simulink model "Rocket_model_Stateflow_testing"  (R2022b)
settings: Solver=VariableStepAuto  StartTime=0.0  StopTime=500  RelTol=1e-3
values from neighbouring files (symbols this model uses):
  GSE_Pipe_Cross_sectional_Area = 7.48    [Rocket_gas_model_setting.m]
  GSE_Pipe_Hydr_Diameter = 2.1    [Rocket_gas_model_setting.m]
  Hose_length = 2    [Rocket_gas_model_setting.m]
  N2_Gas_Tank_Diameter = 0.229    [Rocket_gas_model_setting.m]
  N2_Gas_Tank_Height = 0.5    [Rocket_gas_model_setting.m]
  N2_Rocket_Tank_Diameter = 0.146    [Rocket_gas_model_setting.m]
  N2_Rocket_Tank_Height = 1.515    [Rocket_gas_model_setting.m]
  Outside_temperature = 20    [Rocket_gas_model_setting.m]
  Rocket_Pipe_Cross_sectional_Area = 2    [Rocket_gas_model_setting.m]
  Rocket_Pipe_Hydr_Diameter = 4    [Rocket_gas_model_setting.m]
  s = struct    [State_Flow_varB_setting.m]
libraries: fl_lib x48, nesl_utility x10, slrealtimeiplib x5
settings Model: Creator=START  LastModifiedBy=START

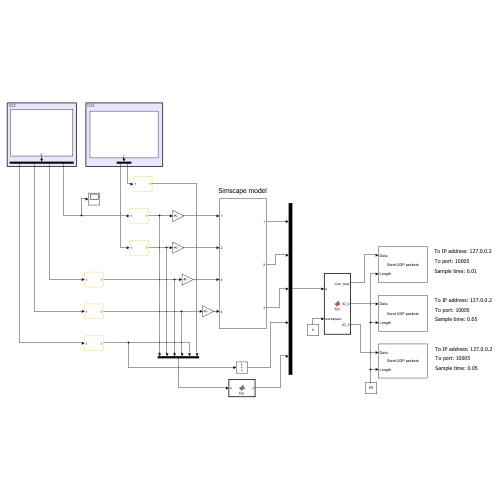
[thumbnail: Simulink's stored preview of the top-level diagram]
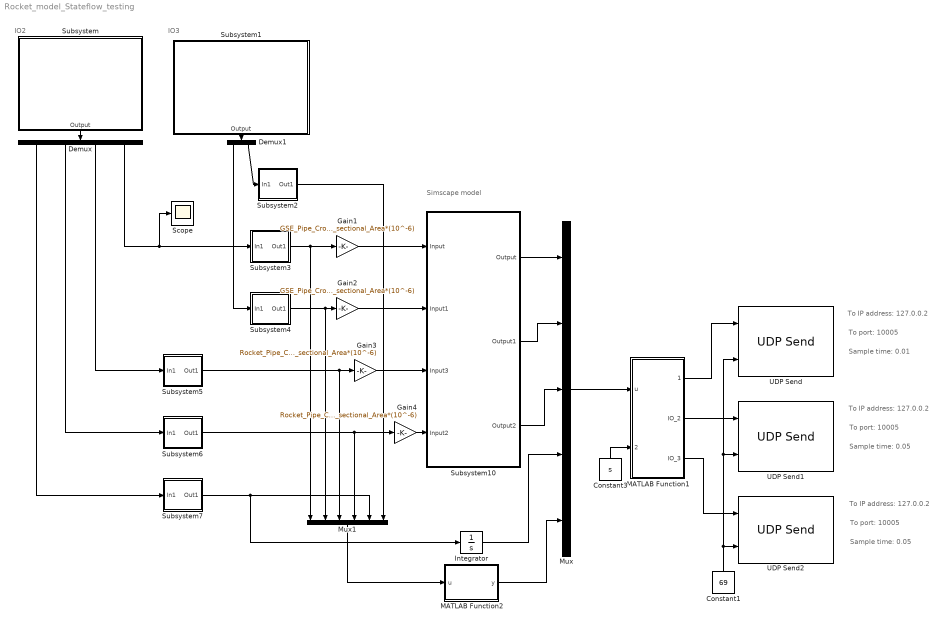
== system Rocket_model_Stateflow_testing ==
  note: Simscape model
  note: To port: 10005
  note: To IP address: 127.0.0.2
  note: IO2
  note: IO3
  note: Sample time: 0.01
  note: Sample time: 0.05
  note: To IP address: 127.0.0.2
  note: To port: 10005
  note: Sample time: 0.05
  note: To IP address: 127.0.0.2
  note: To port: 10005
  Constant1 : Constant  Value=69
  Constant3 : Constant  Value=s  OutDataTypeStr=Bus: s_bus
  Demux : Demux
  Demux1 : Demux  Outputs=2
  Gain1 : Gain  Gain=GSE_Pipe_Cross_sectional_Area*(10^-6)
  Gain2 : Gain  Gain=GSE_Pipe_Cross_sectional_Area*(10^-6)
  Gain3 : Gain  Gain=Rocket_Pipe_Cross_sectional_Area*(10^-6)
  Gain4 : Gain  Gain=Rocket_Pipe_Cross_sectional_Area*(10^-6)
  Integrator : Integrator
  MATLAB Function1 : MATLAB Function  TreatAsAtomicUnit=on
  MATLAB Function2 : MATLAB Function  TreatAsAtomicUnit=on
  Mux : Mux  Inputs=5
  Mux1 : Mux  Inputs=6
  Scope : Scope
  Subsystem : Subsystem
  Subsystem1 : Subsystem
  Subsystem10 : Subsystem
  Subsystem2 : Subsystem
  Subsystem3 : Subsystem
  Subsystem4 : Subsystem
  Subsystem5 : Subsystem
  Subsystem6 : Subsystem
  Subsystem7 : Subsystem
  UDP Send : slrealtimeiplib/UDP Send  useHostTargetConn=off  toAddress=UDP_GSE_receive_local_IP  toPort=UDP_GSE_receive_local_PORT  sampleTime=UDP_GSE_Curr_loop_receive_sample_time  enableMessage=off
  UDP Send1 : slrealtimeiplib/UDP Send  useHostTargetConn=off  toAddress=UDP_GSE_receive_local_IP  toPort=UDP_GSE_receive_local_PORT  sampleTime=UDP_GSE_IO_receive_sample_time  enableMessage=off
  UDP Send2 : slrealtimeiplib/UDP Send  useHostTargetConn=off  toAddress=UDP_GSE_receive_local_IP  toPort=UDP_GSE_receive_local_PORT  sampleTime=UDP_GSE_IO_receive_sample_time  enableMessage=off
  wires:
  Subsystem10/1(Output) -> Mux/1
  Subsystem10/2(Output1) -> Mux/2
  Mux/1 -> MATLAB Function1/1(u)
  Constant1/1 -> UDP Send1/2, UDP Send/2, UDP Send2/2
  Subsystem10/3(Output2) -> Mux/3
  Demux/3 -> Subsystem5/1(In1)
  Subsystem3/1(Out1) -> Gain1/1, Mux1/1
  Subsystem4/1(Out1) -> Gain2/1, Mux1/2
  Subsystem5/1(Out1) -> Gain3/1, Mux1/3
  Demux/2 -> Subsystem6/1(In1)
  Constant3/1 -> MATLAB Function1/2(workspace)
  Subsystem6/1(Out1) -> Gain4/1, Mux1/4
  MATLAB Function2/1(y) -> Mux/5
  Mux1/1 -> MATLAB Function2/1(u)
  MATLAB Function1/1(Curr_loop) -> UDP Send/1
  MATLAB Function1/2(IO_2) -> UDP Send1/1
  MATLAB Function1/3(IO_3) -> UDP Send2/1
  Subsystem7/1(Out1) -> Mux1/5, Integrator/1
  Integrator/1 -> Mux/4
  Subsystem/1(Output) -> Demux/1
  Demux/1 -> Subsystem7/1(In1)
  Demux/4 -> Scope/1, Subsystem3/1(In1)
  Subsystem1/1(Output) -> Demux1/1
  Demux1/1 -> Subsystem4/1(In1)
  Demux1/2 -> Subsystem2/1(In1)
  Subsystem2/1(Out1) -> Mux1/6
  Gain1/1 -> Subsystem10/1(Input)
  Gain2/1 -> Subsystem10/2(Input1)
  Gain3/1 -> Subsystem10/3(Input3)
  Gain4/1 -> Subsystem10/4(Input2)

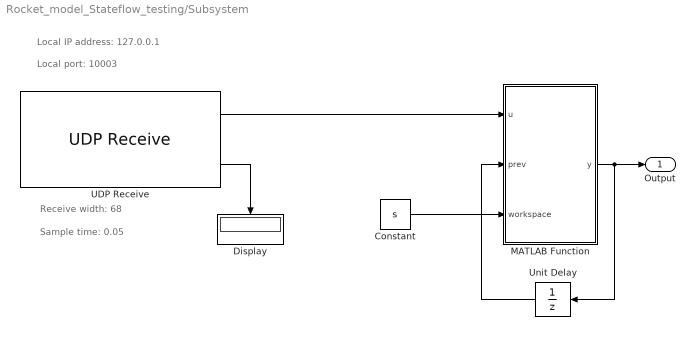
== system Rocket_model_Stateflow_testing/Subsystem ==
  note: Local IP address: 127.0.0.1
  note: Local port: 10003
  note: Receive width: 68
  note: Sample time: 0.05
  Constant : Constant  Value=s  OutDataTypeStr=Bus: s_bus
  Display : Display
  MATLAB Function : MATLAB Function  TreatAsAtomicUnit=on
  UDP Receive : slrealtimeiplib/UDP Receive  useHostTargetConn=off  ipAddress=UDP_GSE_send_to_IP  localPort=IO_card_2_port  rcvWidth=UDP_GSE_send_packet_length  rcvFmAny=on  fmAddress='10.10.10.10'  sampleTime=UDP_GSE_IO_receive_sample_time  enableMessage=off  maxPackets=1
  Unit Delay : UnitDelay  SampleTime=-1  HasFrameUpgradeWarning=on
  Output : Outport
  wires:
  UDP Receive/1 -> MATLAB Function/1(u)
  MATLAB Function/1(y) -> Output/1, Unit Delay/1
  Constant/1 -> MATLAB Function/3(workspace)
  UDP Receive/2 -> Display/1
  Unit Delay/1 -> MATLAB Function/2(prev)

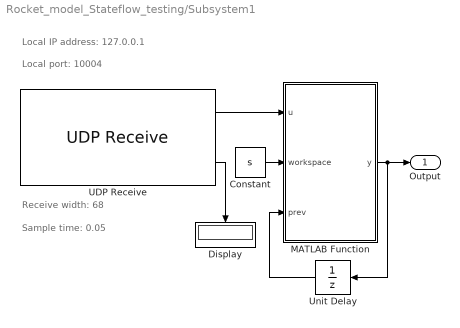
== system Rocket_model_Stateflow_testing/Subsystem1 ==
  note: Local IP address: 127.0.0.1
  note: Local port: 10004
  note: Receive width: 68
  note: Sample time: 0.05
  Constant : Constant  Value=s  OutDataTypeStr=Bus: s_bus
  Display : Display
  MATLAB Function : MATLAB Function  TreatAsAtomicUnit=on
  UDP Receive : slrealtimeiplib/UDP Receive  useHostTargetConn=off  ipAddress=UDP_GSE_send_to_IP  localPort=IO_card_3_port  rcvWidth=UDP_GSE_send_packet_length  rcvFmAny=on  fmAddress='10.10.10.10'  sampleTime=UDP_GSE_IO_receive_sample_time  enableMessage=off  maxPackets=1
  Unit Delay : UnitDelay  InitialCondition=[0,0]  SampleTime=-1  HasFrameUpgradeWarning=on
  Output : Outport
  wires:
  UDP Receive/1 -> MATLAB Function/1(u)
  MATLAB Function/1(y) -> Output/1, Unit Delay/1
  Constant/1 -> MATLAB Function/2(workspace)
  UDP Receive/2 -> Display/1
  Unit Delay/1 -> MATLAB Function/3(prev)

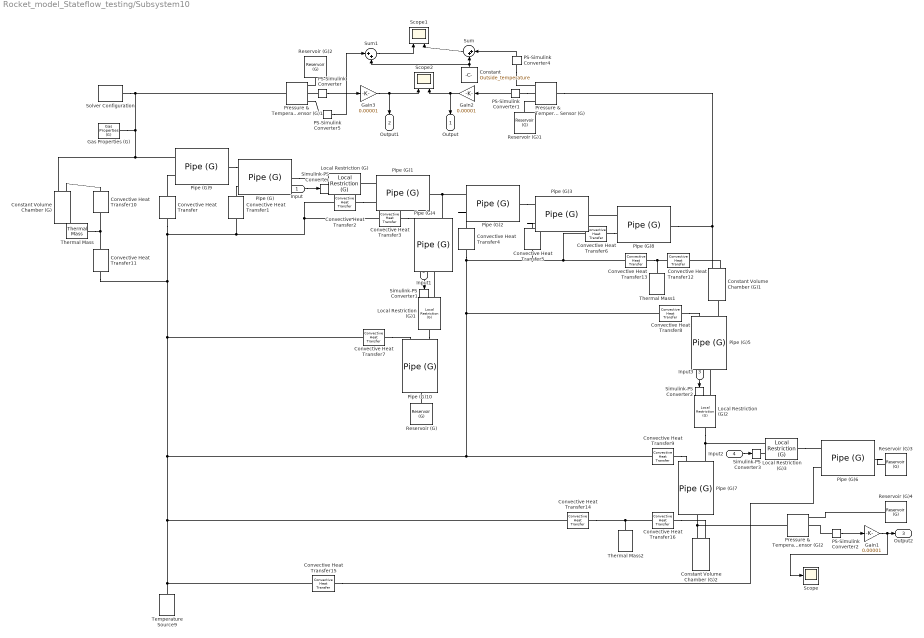
== system Rocket_model_Stateflow_testing/Subsystem10 ==
  Input : Inport
  Input1 : Inport  Port=2
  Input3 : Inport  Port=3
  Input2 : Inport  Port=4
  Constant : Constant  Value=Outside_temperature
  Constant Volume Chamber (G) : fl_lib/Gas/Elements/Constant Volume Chamber (G)  volume=N2_Gas_Tank_Volume m^3  num_ports=foundation.enum.num_ports.one  area_A=0.001 m^2  area_B=0.01 m^2  area_C=0.01 m^2  area_D=0.01 m^2  p_I_specify=on  p_I_priority=High  p_I=N2_Gas_Tank_Pressure bar  p_I_nominal_specify=off  p_I_nominal_unit=MPa  p_I_nominal_value=1  T_I_specify=on  T_I_priority=Low  T_I=Outside_temperature degC  T_I_nominal_specify=off  T_I_nominal_unit=K  T_I_nominal_value=293  rho_chamber_specify=off  rho_chamber_priority=None  rho_chamber=1.2 kg/m^3  rho_chamber_nominal_specify=off  rho_chamber_nominal_unit=kg/m^3  rho_chamber_nominal_value=1
      settings: InternalSimscapePortConfiguration="{\"Bottom\":[],\"Left\":[{\"id\":\"A\",\"label\":\"A\",\"type\":\"foundation.gas.gas\"},{\"id\":\"H\",\"label\":\"H\",\"type\":\"foundation.thermal.thermal\"}],\"Right\":[],\"Top\":[]}"
  Constant Volume Chamber (G)1 : fl_lib/Gas/Elements/Constant Volume Chamber (G)  volume=N2_Rocket_Tank_Volume m^3  num_ports=foundation.enum.num_ports.two  area_A=0.001 m^2  area_B=0.001 m^2  area_C=0.01 m^2  area_D=0.01 m^2  p_I_specify=on  p_I_priority=High  p_I=1 bar  p_I_nominal_specify=off  p_I_nominal_unit=MPa  p_I_nominal_value=1  T_I_specify=on  T_I_priority=Low  T_I=Outside_temperature degC  T_I_nominal_specify=off  T_I_nominal_unit=K  T_I_nominal_value=320  rho_chamber_specify=off  rho_chamber_priority=None  rho_chamber=1.2 kg/m^3  rho_chamber_nominal_specify=off  rho_chamber_nominal_unit=kg/m^3  rho_chamber_nominal_value=1
      settings: InternalSimscapePortConfiguration="{\"Bottom\":[],\"Left\":[{\"id\":\"A\",\"label\":\"A\",\"type\":\"foundation.gas.gas\"},{\"id\":\"H\",\"label\":\"H\",\"type\":\"foundation.thermal.thermal\"}],\"Right\":[{\"id\":\"B\",\"label\":\"B\",\"type\":\"foundation.gas.gas\"}],\"Top\":[]}"
  Constant Volume Chamber (G)2 : fl_lib/Gas/Elements/Constant Volume Chamber (G)  volume=N2O_Rocket_Tank_Volume m^3  num_ports=foundation.enum.num_ports.one  area_A=0.001 m^2  area_B=0.001 m^2  area_C=0.01 m^2  area_D=0.01 m^2  p_I_specify=on  p_I_priority=High  p_I=1 bar  p_I_nominal_specify=off  p_I_nominal_unit=MPa  p_I_nominal_value=1  T_I_specify=on  T_I_priority=Low  T_I=Outside_temperature degC  T_I_nominal_specify=off  T_I_nominal_unit=K  T_I_nominal_value=320  rho_chamber_specify=off  rho_chamber_priority=None  rho_chamber=1.2 kg/m^3  rho_chamber_nominal_specify=off  rho_chamber_nominal_unit=kg/m^3  rho_chamber_nominal_value=1
      settings: InternalSimscapePortConfiguration="{\"Bottom\":[],\"Left\":[{\"id\":\"A\",\"label\":\"A\",\"type\":\"foundation.gas.gas\"},{\"id\":\"H\",\"label\":\"H\",\"type\":\"foundation.thermal.thermal\"}],\"Right\":[],\"Top\":[]}"
  Convective Heat Transfer : fl_lib/Thermal/Thermal Elements/Convective Heat Transfer  thermal_type=foundation.enum.constant_variable.constant  area=GSE_Pipe_Hydr_Diameter*(Hose_length*1000) mm^2  heat_tr_coeff=15 W/(K*m^2)  min_heat_tr_coeff=1e-3 W/(K*m^2)  T_specify=off  T_priority=None  T=0 K  T_nominal_specify=off  T_nominal_unit=K  T_nominal_value=1  Q_specify=off  Q_priority=None  Q=0 W  Q_nominal_specify=off  Q_nominal_unit=W  Q_nominal_value=1
  Convective Heat Transfer1 : fl_lib/Thermal/Thermal Elements/Convective Heat Transfer  thermal_type=foundation.enum.constant_variable.constant  area=GSE_Pipe_Hydr_Diameter*(0.3*1000) mm^2  heat_tr_coeff=15 W/(K*m^2)  min_heat_tr_coeff=1e-3 W/(K*m^2)  T_specify=off  T_priority=None  T=0 K  T_nominal_specify=off  T_nominal_unit=K  T_nominal_value=1  Q_specify=off  Q_priority=None  Q=0 W  Q_nominal_specify=off  Q_nominal_unit=W  Q_nominal_value=1
  Convective Heat Transfer10 : fl_lib/Thermal/Thermal Elements/Convective Heat Transfer  thermal_type=foundation.enum.constant_variable.constant  area="N2_Gas_Tank_Diameter*N2_Gas_Tank_Height  m^2"  heat_tr_coeff=15 W/(K*m^2)  min_heat_tr_coeff=1e-3 W/(K*m^2)  T_specify=off  T_priority=None  T=0 K  T_nominal_specify=off  T_nominal_unit=K  T_nominal_value=1  Q_specify=off  Q_priority=None  Q=0 W  Q_nominal_specify=off  Q_nominal_unit=W  Q_nominal_value=1
  Convective Heat Transfer11 : fl_lib/Thermal/Thermal Elements/Convective Heat Transfer  thermal_type=foundation.enum.constant_variable.constant  area="N2_Gas_Tank_Diameter*N2_Gas_Tank_Height  m^2"  heat_tr_coeff=15 W/(K*m^2)  min_heat_tr_coeff=1e-3 W/(K*m^2)  T_specify=off  T_priority=None  T=0 K  T_nominal_specify=off  T_nominal_unit=K  T_nominal_value=1  Q_specify=off  Q_priority=None  Q=0 W  Q_nominal_specify=off  Q_nominal_unit=W  Q_nominal_value=1
  Convective Heat Transfer12 : fl_lib/Thermal/Thermal Elements/Convective Heat Transfer  thermal_type=foundation.enum.constant_variable.constant  area="N2_Rocket_Tank_Diameter*N2_Rocket_Tank_Height  m^2"  heat_tr_coeff=15 W/(K*m^2)  min_heat_tr_coeff=1e-3 W/(K*m^2)  T_specify=off  T_priority=None  T=0 K  T_nominal_specify=off  T_nominal_unit=K  T_nominal_value=1  Q_specify=off  Q_priority=None  Q=0 W  Q_nominal_specify=off  Q_nominal_unit=W  Q_nominal_value=1
  Convective Heat Transfer13 : fl_lib/Thermal/Thermal Elements/Convective Heat Transfer  thermal_type=foundation.enum.constant_variable.constant  area="N2_Rocket_Tank_Diameter*N2_Rocket_Tank_Height  m^2"  heat_tr_coeff=15 W/(K*m^2)  min_heat_tr_coeff=1e-3 W/(K*m^2)  T_specify=off  T_priority=None  T=0 K  T_nominal_specify=off  T_nominal_unit=K  T_nominal_value=1  Q_specify=off  Q_priority=None  Q=0 W  Q_nominal_specify=off  Q_nominal_unit=W  Q_nominal_value=1
  Convective Heat Transfer{9,14..16} (4 alike) : fl_lib/Thermal/Thermal Elements/Convective Heat Transfer  thermal_type=foundation.enum.constant_variable.constant  area=Rocket_Pipe_Hydr_Diameter*(0.2*1000) mm^2  heat_tr_coeff=15 W/(K*m^2)  min_heat_tr_coeff=1e-3 W/(K*m^2)  T_specify=off  T_priority=None  T=0 K  T_nominal_specify=off  T_nominal_unit=K  T_nominal_value=1  Q_specify=off  Q_priority=None  Q=0 W  Q_nominal_specify=off  Q_nominal_unit=W  Q_nominal_value=1
  Convective Heat Transfer{2..3,6..7} (4 alike) : fl_lib/Thermal/Thermal Elements/Convective Heat Transfer  thermal_type=foundation.enum.constant_variable.constant  area=GSE_Pipe_Hydr_Diameter*(0.1*1000) mm^2  heat_tr_coeff=15 W/(K*m^2)  min_heat_tr_coeff=1e-3 W/(K*m^2)  T_specify=off  T_priority=None  T=0 K  T_nominal_specify=off  T_nominal_unit=K  T_nominal_value=1  Q_specify=off  Q_priority=None  Q=0 W  Q_nominal_specify=off  Q_nominal_unit=W  Q_nominal_value=1
  Convective Heat Transfer4 : fl_lib/Thermal/Thermal Elements/Convective Heat Transfer  thermal_type=foundation.enum.constant_variable.constant  area=GSE_Pipe_Hydr_Diameter*(0.2*1000) mm^2  heat_tr_coeff=15 W/(K*m^2)  min_heat_tr_coeff=1e-3 W/(K*m^2)  T_specify=off  T_priority=None  T=0 K  T_nominal_specify=off  T_nominal_unit=K  T_nominal_value=1  Q_specify=off  Q_priority=None  Q=0 W  Q_nominal_specify=off  Q_nominal_unit=W  Q_nominal_value=1
  Convective Heat Transfer5 : fl_lib/Thermal/Thermal Elements/Convective Heat Transfer  thermal_type=foundation.enum.constant_variable.constant  area=GSE_Pipe_Hydr_Diameter*(Hose_length*1000) mm^2  heat_tr_coeff=15 W/(K*m^2)  min_heat_tr_coeff=1e-3 W/(K*m^2)  T_specify=off  T_priority=None  T=0 K  T_nominal_specify=off  T_nominal_unit=K  T_nominal_value=1  Q_specify=off  Q_priority=None  Q=0 W  Q_nominal_specify=off  Q_nominal_unit=W  Q_nominal_value=1
  Convective Heat Transfer8 : fl_lib/Thermal/Thermal Elements/Convective Heat Transfer  thermal_type=foundation.enum.constant_variable.constant  area=Rocket_Pipe_Hydr_Diameter*(0.1*1000) mm^2  heat_tr_coeff=15 W/(K*m^2)  min_heat_tr_coeff=1e-3 W/(K*m^2)  T_specify=off  T_priority=None  T=0 K  T_nominal_specify=off  T_nominal_unit=K  T_nominal_value=1  Q_specify=off  Q_priority=None  Q=0 W  Q_nominal_specify=off  Q_nominal_unit=W  Q_nominal_value=1
  Gain1 : Gain  Gain=0.00001
  Gain2 : Gain  Gain=0.00001
  Gain3 : Gain  Gain=0.00001
  Gas Properties (G) : fl_lib/Gas/Utilities/Gas Properties (G)  gas_spec=foundation.enum.gas_spec.real_gas  R=0.287 kJ/(K*kg)  Z=1  T_ref=293.15 K  h_ref=420 kJ/kg  cp_ref=1 kJ/(K*kg)  mu_ref=18 s*uPa  k_ref=26 mW/(K*m)  T_TLU1=[150 : 10 : 200, 250 : 50 : 1000, 1500, 2000]' K  h_TLU1=[275.264783730547; 285.377054177734; 295.474578903607; 305.560871069627; 315.638490783961; 325.709373787179; 376.008033649461; 426.297784741196; 476.678788323875; 527.253890684429; 578.12722735187; 629.395040865183; 681.137690131207; 733.415442873049; 786.267894376777; 839.715851152006; 893.764459999509; 948.406676876931; 1003.62653219711; 1059.40193232821; 1115.70691941005; 1172.51341226958; 1762.18512007361; 2377.14064127409] kJ/kg  cp_TLU1=[1.01211492398124; 1.01042105529234; 1.00914159006373; 1.00815898273273; 1.00739688341918; 1.00680484569075; 1.00554191216852; 1.00637389921747; 1.0092105862442; 1.01414404435034; 1.02111299587909; 1.02986878923959; 1.04003820504128; 1.05120320041448; 1.06296312852444; 1.07497111709439; 1.08694865668905; 1.0986858495625; 1.11003396604319; 1.12089493621399; 1.13121051694521; 1.14095251451866; 1.21001953144; 1.24628356718428] kJ/(K*kg)  mu_TLU1=[10.3766056544352; 10.9908682444892; 11.5932000841352; 12.1841060353213; 12.764067709023; 13.3335437107148; 16.038149065057; 18.5373404836509; 20.8671495114253; 23.0554226800681; 25.1239717991959; 27.0901379793485; 28.96790749834; 30.7687111230031; 32.5020036481173; 34.17569027566; 35.7964450415303; 37.3699520751368; 38.9010908824946; 40.3940804368247; 41.8525925389218; 43.279841956487; 56.3254722619962; 68.068290080945] s*uPa  k_TLU1=[14.1517155766309; 15.0474512994325; 15.9300520513026; 16.7998749295306; 17.6573089963228; 18.5027588910197; 22.5644026699512; 26.384465676638; 30.0032801168886; 33.4532006033488; 36.7600619429332; 39.9446251241844; 43.0237448740114; 46.0112537033799; 48.9186234516389; 51.7554617696538; 54.5298878921773; 57.2488200454925; 59.9181976996146; 62.5431553064749; 65.128159527924; 67.6771186900213; 91.7815514375552; 114.486299090693] mW/(K*m)  T_TLU2=T K  p_TLU2=P bar  rho_TLU2=Rho kg/m^3  s_TLU2=S kJ/(K*kg)  h_TLU2=H kJ/kg  cp_TLU2=Cp kJ/(K*kg)  mu_TLU2=mu s*uPa  k_TLU2=k mW/(K*m)  beta_TLU2=bulk_modulus Pa  alpha_TLU2=isobaric_thermal_expansion_coeff 1/K  T_min_perfect=1 K  T_max_perfect=inf K  p_min_perfect=1 Pa  p_max_perfect=inf MPa  T_range_flag=foundation.enum.T_range_G.from_props  T_min_semiperfect=150 K  T_max_semiperfect=2000 K  p_min_semiperfect=1 Pa  p_max_semiperfect=inf MPa  pT_region_flag=foundation.enum.pT_region_G.min_max  pT_validity_TLU2=ones(24, 20)  T_min_real=150 K  T_max_real=2000 K  p_min_real=0.00001 bar  p_max_real=1000 bar  p_atm=0.101325 MPa  Mach_rev=0.001
  Local Restriction (G) : fl_lib/Gas/Elements/Local Restriction (G)  restriction_type=foundation.enum.restriction_type.variable  restriction_area=1e-3 m^2  min_area=1e-10 m^2  max_area=GSE_Pipe_Cross_sectional_Area mm^2  area=GSE_Pipe_Cross_sectional_Area+0.01 mm^2  Cd=0.64  B_lam=0.999
      settings: InternalSimscapePortConfiguration="{\"Bottom\":[],\"Left\":[{\"id\":\"A\",\"label\":\"A\",\"type\":\"foundation.gas.gas\"},{\"id\":\"area_in\",\"label\":\"AR\",\"type\":\"input\"}],\"Right\":[{\"id\":\"B\",\"label\":\"B\",\"type\":\"foundation.gas.gas\"}],\"Top\":[]}"
  Local Restriction (G)1 : fl_lib/Gas/Elements/Local Restriction (G)  restriction_type=foundation.enum.restriction_type.variable  restriction_area=1e-3 m^2  min_area=1e-10 m^2  max_area=GSE_Pipe_Cross_sectional_Area mm^2  area=GSE_Pipe_Cross_sectional_Area+0.01 mm^2  Cd=0.64  B_lam=0.999
      settings: InternalSimscapePortConfiguration="{\"Bottom\":[],\"Left\":[{\"id\":\"A\",\"label\":\"A\",\"type\":\"foundation.gas.gas\"},{\"id\":\"area_in\",\"label\":\"AR\",\"type\":\"input\"}],\"Right\":[{\"id\":\"B\",\"label\":\"B\",\"type\":\"foundation.gas.gas\"}],\"Top\":[]}"
  Local Restriction (G)2 : fl_lib/Gas/Elements/Local Restriction (G)  restriction_type=foundation.enum.restriction_type.variable  restriction_area=1e-3 m^2  min_area=1e-10 m^2  max_area=Rocket_Pipe_Cross_sectional_Area mm^2  area=Rocket_Pipe_Cross_sectional_Area+0.01 mm^2  Cd=0.64  B_lam=0.999
      settings: InternalSimscapePortConfiguration="{\"Bottom\":[],\"Left\":[{\"id\":\"A\",\"label\":\"A\",\"type\":\"foundation.gas.gas\"},{\"id\":\"area_in\",\"label\":\"AR\",\"type\":\"input\"}],\"Right\":[{\"id\":\"B\",\"label\":\"B\",\"type\":\"foundation.gas.gas\"}],\"Top\":[]}"
  Local Restriction (G)3 : fl_lib/Gas/Elements/Local Restriction (G)  restriction_type=foundation.enum.restriction_type.variable  restriction_area=1e-3 m^2  min_area=1e-10 m^2  max_area=Rocket_Pipe_Cross_sectional_Area mm^2  area=Rocket_Pipe_Cross_sectional_Area+0.01 mm^2  Cd=0.64  B_lam=0.999
      settings: InternalSimscapePortConfiguration="{\"Bottom\":[],\"Left\":[{\"id\":\"A\",\"label\":\"A\",\"type\":\"foundation.gas.gas\"},{\"id\":\"area_in\",\"label\":\"AR\",\"type\":\"input\"}],\"Right\":[{\"id\":\"B\",\"label\":\"B\",\"type\":\"foundation.gas.gas\"}],\"Top\":[]}"
  PS-Simulink Converter{,1..2,4..5} (5 alike) : nesl_utility/PS-Simulink Converter  PhysicalDomain=network_engine_domain  SubClassName=ps_output  LeftPortType=input  RightPortType=output  PseudoPeriodic=off  Frequencies=[]  VectorFormat=inherit  Unit=inherit  AffineConversion=off
  Pipe (G) : fl_lib/Gas/Elements/Pipe (G)  length=0.3 m  area=GSE_Pipe_Cross_sectional_Area mm^2  Dh=GSE_Pipe_Hydr_Diameter mm  length_add=0.1 m  roughness=15e-6 m  Re_lam=2000  Re_tur=4000  shape_factor=64  Nu_lam=3.66  p_I_specify=off  p_I_priority=High  p_I=0.101325 MPa  p_I_nominal_specify=off  p_I_nominal_unit=MPa  p_I_nominal_value=1  T_I_specify=on  T_I_priority=Low  T_I=Outside_temperature degC  T_I_nominal_specify=off  T_I_nominal_unit=K  T_I_nominal_value=1  rho_pipe_specify=off  rho_pipe_priority=None  rho_pipe=1.2 kg/m^3  rho_pipe_nominal_specify=off  rho_pipe_nominal_unit=kg/m^3  rho_pipe_nominal_value=1
  Pipe (G)1 : fl_lib/Gas/Elements/Pipe (G)  length=0.1 m  area=GSE_Pipe_Cross_sectional_Area mm^2  Dh=GSE_Pipe_Hydr_Diameter mm  length_add=0.1 m  roughness=15e-6 m  Re_lam=2000  Re_tur=4000  shape_factor=64  Nu_lam=3.66  p_I_specify=off  p_I_priority=High  p_I=0.101325 MPa  p_I_nominal_specify=off  p_I_nominal_unit=MPa  p_I_nominal_value=1  T_I_specify=on  T_I_priority=Low  T_I=Outside_temperature degC  T_I_nominal_specify=off  T_I_nominal_unit=K  T_I_nominal_value=1  rho_pipe_specify=off  rho_pipe_priority=None  rho_pipe=1.2 kg/m^3  rho_pipe_nominal_specify=off  rho_pipe_nominal_unit=kg/m^3  rho_pipe_nominal_value=1
  Pipe (G)10 : fl_lib/Gas/Elements/Pipe (G)  length=0.1 m  area=GSE_Pipe_Cross_sectional_Area mm^2  Dh=GSE_Pipe_Hydr_Diameter mm  length_add=0.1 m  roughness=15e-6 m  Re_lam=2000  Re_tur=4000  shape_factor=64  Nu_lam=3.66  p_I_specify=off  p_I_priority=High  p_I=0.101325 MPa  p_I_nominal_specify=off  p_I_nominal_unit=MPa  p_I_nominal_value=1  T_I_specify=on  T_I_priority=Low  T_I=Outside_temperature degC  T_I_nominal_specify=off  T_I_nominal_unit=K  T_I_nominal_value=1  rho_pipe_specify=off  rho_pipe_priority=None  rho_pipe=1.2 kg/m^3  rho_pipe_nominal_specify=off  rho_pipe_nominal_unit=kg/m^3  rho_pipe_nominal_value=1
  Pipe (G)2 : fl_lib/Gas/Elements/Pipe (G)  length=0.2 m  area=GSE_Pipe_Cross_sectional_Area mm^2  Dh=GSE_Pipe_Hydr_Diameter mm  length_add=0.1 m  roughness=15e-6 m  Re_lam=2000  Re_tur=4000  shape_factor=64  Nu_lam=3.66  p_I_specify=off  p_I_priority=High  p_I=0.101325 MPa  p_I_nominal_specify=off  p_I_nominal_unit=MPa  p_I_nominal_value=1  T_I_specify=on  T_I_priority=Low  T_I=Outside_temperature degC  T_I_nominal_specify=off  T_I_nominal_unit=K  T_I_nominal_value=1  rho_pipe_specify=off  rho_pipe_priority=None  rho_pipe=1.2 kg/m^3  rho_pipe_nominal_specify=off  rho_pipe_nominal_unit=kg/m^3  rho_pipe_nominal_value=1
  Pipe (G)3 : fl_lib/Gas/Elements/Pipe (G)  length=Hose_length m  area=GSE_Pipe_Cross_sectional_Area mm^2  Dh=GSE_Pipe_Hydr_Diameter mm  length_add=0.1 m  roughness=15e-6 m  Re_lam=2000  Re_tur=4000  shape_factor=64  Nu_lam=3.66  p_I_specify=off  p_I_priority=High  p_I=0.101325 MPa  p_I_nominal_specify=off  p_I_nominal_unit=MPa  p_I_nominal_value=1  T_I_specify=on  T_I_priority=Low  T_I=Outside_temperature degC  T_I_nominal_specify=off  T_I_nominal_unit=K  T_I_nominal_value=1  rho_pipe_specify=off  rho_pipe_priority=None  rho_pipe=1.2 kg/m^3  rho_pipe_nominal_specify=off  rho_pipe_nominal_unit=kg/m^3  rho_pipe_nominal_value=1
  Pipe (G)4 : fl_lib/Gas/Elements/Pipe (G)  length=0.4 m  area=GSE_Pipe_Cross_sectional_Area mm^2  Dh=GSE_Pipe_Hydr_Diameter mm  length_add=0.1 m  roughness=15e-6 m  Re_lam=2000  Re_tur=4000  shape_factor=64  Nu_lam=3.66  p_I_specify=off  p_I_priority=High  p_I=0.101325 MPa  p_I_nominal_specify=off  p_I_nominal_unit=MPa  p_I_nominal_value=1  T_I_specify=on  T_I_priority=Low  T_I=Outside_temperature degC  T_I_nominal_specify=off  T_I_nominal_unit=K  T_I_nominal_value=1  rho_pipe_specify=off  rho_pipe_priority=None  rho_pipe=1.2 kg/m^3  rho_pipe_nominal_specify=off  rho_pipe_nominal_unit=kg/m^3  rho_pipe_nominal_value=1
  Pipe (G)5 : fl_lib/Gas/Elements/Pipe (G)  length=0.1 m  area=Rocket_Pipe_Cross_sectional_Area mm^2  Dh=Rocket_Pipe_Hydr_Diameter mm  length_add=0.1 m  roughness=15e-6 m  Re_lam=2000  Re_tur=4000  shape_factor=64  Nu_lam=3.66  p_I_specify=off  p_I_priority=High  p_I=0.101325 MPa  p_I_nominal_specify=off  p_I_nominal_unit=MPa  p_I_nominal_value=1  T_I_specify=on  T_I_priority=Low  T_I=Outside_temperature degC  T_I_nominal_specify=off  T_I_nominal_unit=K  T_I_nominal_value=1  rho_pipe_specify=off  rho_pipe_priority=None  rho_pipe=1.2 kg/m^3  rho_pipe_nominal_specify=off  rho_pipe_nominal_unit=kg/m^3  rho_pipe_nominal_value=1
  Pipe (G)6 : fl_lib/Gas/Elements/Pipe (G)  length=0.1 m  area=Rocket_Pipe_Cross_sectional_Area mm^2  Dh=Rocket_Pipe_Hydr_Diameter mm  length_add=0.1 m  roughness=15e-6 m  Re_lam=2000  Re_tur=4000  shape_factor=64  Nu_lam=3.66  p_I_specify=off  p_I_priority=High  p_I=0.101325 MPa  p_I_nominal_specify=off  p_I_nominal_unit=MPa  p_I_nominal_value=1  T_I_specify=on  T_I_priority=Low  T_I=Outside_temperature degC  T_I_nominal_specify=off  T_I_nominal_unit=K  T_I_nominal_value=1  rho_pipe_specify=off  rho_pipe_priority=None  rho_pipe=1.2 kg/m^3  rho_pipe_nominal_specify=off  rho_pipe_nominal_unit=kg/m^3  rho_pipe_nominal_value=1
  Pipe (G)7 : fl_lib/Gas/Elements/Pipe (G)  length=0.2 m  area=Rocket_Pipe_Cross_sectional_Area mm^2  Dh=Rocket_Pipe_Hydr_Diameter mm  length_add=0.1 m  roughness=15e-6 m  Re_lam=2000  Re_tur=4000  shape_factor=64  Nu_lam=3.66  p_I_specify=off  p_I_priority=High  p_I=0.101325 MPa  p_I_nominal_specify=off  p_I_nominal_unit=MPa  p_I_nominal_value=1  T_I_specify=on  T_I_priority=Low  T_I=Outside_temperature degC  T_I_nominal_specify=off  T_I_nominal_unit=K  T_I_nominal_value=1  rho_pipe_specify=off  rho_pipe_priority=None  rho_pipe=1.2 kg/m^3  rho_pipe_nominal_specify=off  rho_pipe_nominal_unit=kg/m^3  rho_pipe_nominal_value=1
  Pipe (G)8 : fl_lib/Gas/Elements/Pipe (G)  length=0.1 m  area=GSE_Pipe_Cross_sectional_Area mm^2  Dh=GSE_Pipe_Hydr_Diameter mm  length_add=0.1 m  roughness=15e-6 m  Re_lam=2000  Re_tur=4000  shape_factor=64  Nu_lam=3.66  p_I_specify=off  p_I_priority=High  p_I=0.101325 MPa  p_I_nominal_specify=off  p_I_nominal_unit=MPa  p_I_nominal_value=1  T_I_specify=on  T_I_priority=Low  T_I=Outside_temperature degC  T_I_nominal_specify=off  T_I_nominal_unit=K  T_I_nominal_value=1  rho_pipe_specify=off  rho_pipe_priority=None  rho_pipe=1.2 kg/m^3  rho_pipe_nominal_specify=off  rho_pipe_nominal_unit=kg/m^3  rho_pipe_nominal_value=1
  Pipe (G)9 : fl_lib/Gas/Elements/Pipe (G)  length=Hose_length m  area=GSE_Pipe_Cross_sectional_Area mm^2  Dh=GSE_Pipe_Hydr_Diameter mm  length_add=0.1 m  roughness=15e-6 m  Re_lam=2000  Re_tur=4000  shape_factor=64  Nu_lam=3.66  p_I_specify=off  p_I_priority=High  p_I=0.101325 MPa  p_I_nominal_specify=off  p_I_nominal_unit=MPa  p_I_nominal_value=1  T_I_specify=on  T_I_priority=Low  T_I=Outside_temperature degC  T_I_nominal_specify=off  T_I_nominal_unit=K  T_I_nominal_value=1  rho_pipe_specify=off  rho_pipe_priority=None  rho_pipe=1.2 kg/m^3  rho_pipe_nominal_specify=off  rho_pipe_nominal_unit=kg/m^3  rho_pipe_nominal_value=1
  Pressure & Temperature Sensor (G) : fl_lib/Gas/Sensors/Pressure & Temperature Sensor (G)
      settings: InternalSimscapePortConfiguration="{\"Bottom\":[],\"Left\":[{\"id\":\"A\",\"label\":\"A\",\"type\":\"foundation.gas.gas\"}],\"Right\":[{\"id\":\"B\",\"label\":\"B\",\"type\":\"foundation.gas.gas\"},{\"id\":\"P\",\"label\":\"P\",\"type\":\"output\"},{\"id\":\"T\",\"label\":\"T\",\"type\":\"output\"}],\"Top\":[]}"
  Pressure & Temperature Sensor (G)1 : fl_lib/Gas/Sensors/Pressure & Temperature Sensor (G)
      settings: InternalSimscapePortConfiguration="{\"Bottom\":[],\"Left\":[{\"id\":\"A\",\"label\":\"A\",\"type\":\"foundation.gas.gas\"}],\"Right\":[{\"id\":\"B\",\"label\":\"B\",\"type\":\"foundation.gas.gas\"},{\"id\":\"P\",\"label\":\"P\",\"type\":\"output\"},{\"id\":\"T\",\"label\":\"T\",\"type\":\"output\"}],\"Top\":[]}"
  Pressure & Temperature Sensor (G)2 : fl_lib/Gas/Sensors/Pressure & Temperature Sensor (G)
      settings: InternalSimscapePortConfiguration="{\"Bottom\":[],\"Left\":[{\"id\":\"A\",\"label\":\"A\",\"type\":\"foundation.gas.gas\"}],\"Right\":[{\"id\":\"B\",\"label\":\"B\",\"type\":\"foundation.gas.gas\"},{\"id\":\"P\",\"label\":\"P\",\"type\":\"output\"},{\"id\":\"T\",\"label\":\"T\",\"type\":\"output\"}],\"Top\":[]}"
  Reservoir (G) : fl_lib/Gas/Elements/Reservoir (G)  pressure_spec=foundation.enum.pressure_spec.atmospheric  reservoir_pressure=0.101325 MPa  reservoir_temperature=Outside_temperature degC  area_A=0.01 m^2
  Reservoir (G)1 : fl_lib/Gas/Elements/Reservoir (G)  pressure_spec=foundation.enum.pressure_spec.specified  reservoir_pressure=0.00001 bar  reservoir_temperature=Outside_temperature degC  area_A=0.01 m^2
  Reservoir (G)2 : fl_lib/Gas/Elements/Reservoir (G)  pressure_spec=foundation.enum.pressure_spec.specified  reservoir_pressure=0.00001 bar  reservoir_temperature=Outside_temperature degC  area_A=0.01 m^2
  Reservoir (G)3 : fl_lib/Gas/Elements/Reservoir (G)  pressure_spec=foundation.enum.pressure_spec.atmospheric  reservoir_pressure=0.101325 MPa  reservoir_temperature=Outside_temperature degC  area_A=0.01 m^2
  Reservoir (G)4 : fl_lib/Gas/Elements/Reservoir (G)  pressure_spec=foundation.enum.pressure_spec.specified  reservoir_pressure=0.00001 bar  reservoir_temperature=Outside_temperature degC  area_A=0.01 m^2
  Scope : Scope
  Scope1 : Scope  NumInputPorts=2
  Scope2 : Scope  NumInputPorts=2
  Simulink-PS Converter{,1..3} (4 alike) : nesl_utility/Simulink-PS Converter  PhysicalDomain=network_engine_domain  SubClassName=ps_input  LeftPortType=input  RightPortType=output  PseudoPeriodic=off  Frequencies=[]  NoiseDistribution=none  NoiseParameters=[]  Unit=1  AffineConversion=off  FilteringAndDerivatives=provide  SimscapeFilterOrder=1  InputFilterTimeConstant=0.001  UdotUserProvided=0
  Solver Configuration : nesl_utility/Solver Configuration  PhysicalDomain=network_engine_domain  SubClassName=solver  LeftPortType=input  RightPortType=generic  Tones=[]  Harmonics=[]  SimulateNoise=off  Profile=off  UseLocalSampling=off  EnableSwitchedLinearOptims=on  FrequencyDomain=off  UseCCode=off  RelTol=0.001  AbsTol=0.001  MinStep=1e-09  ToWorkspace=off  RevertToSquareIcSolve=off  NumHomotopyIterations=100  PhasorMode=off  PhasorModeNumHarmonics=1  ConsistencySolver=NEWTON_XTOL_AFTER_FTOL  IndexReductionMethod=DerivativeReplacement  DoDC=off  ResidualTolerance=1e-09  ConsistencyTolSource=GLOBAL  ConsistencyAbsTol=0.001  ConsistencyRelTol=0.001  ConsistencyTolFactor=0.001  UseLocalSolver=off  LocalSolverChoice=NE_BACKWARD_EULER_ADVANCER  ResolveIndetEquations=on  FunctionEvalNumThread=1  LocalSolverSampleTime=0.001  DoFixedCost=off  MaxNonlinIter=3  MaxModeIter=2  ComputeImpulses=off  ImpulseIterations=2  LinearAlgebra=auto  LinearAlgebraNumThread=0  EquationFormulation=NE_TIME_EF  DelaysMemoryBudget=1024  AutomaticFiltering=on  FilteringTimeConstant=0.001  PartitionStorageMethod=AS_NEEDED  PartitionMemoryBudget=1024  PartitionMethod=ROBUST
  Sum : Sum  Inputs=|++
  Sum1 : Sum  Inputs=|++
  Temperature Source9 : fl_lib/Thermal/Thermal Sources/Temperature Source  temperature=Outside_temperature degC
  Thermal Mass : fl_lib/Thermal/Thermal Elements/Thermal Mass  mass=N2_Gas_Tank_Mass kg  sp_heat=N2_Gas_Tank_C J/(K*kg)  num_ports=foundation.enum.numPorts2.one  T_specify=on  T_priority=Low  T=Outside_temperature degC  T_nominal_specify=off  T_nominal_unit=K  T_nominal_value=1  Q_specify=off  Q_priority=None  Q=0 W  Q_nominal_specify=off  Q_nominal_unit=W  Q_nominal_value=1
  Thermal Mass1 : fl_lib/Thermal/Thermal Elements/Thermal Mass  mass=N2_Rocket_Tank_Mass kg  sp_heat=N2_Rocket_Tank_C J/(K*kg)  num_ports=foundation.enum.numPorts2.one  T_specify=on  T_priority=Low  T=Outside_temperature degC  T_nominal_specify=off  T_nominal_unit=K  T_nominal_value=1  Q_specify=off  Q_priority=None  Q=0 W  Q_nominal_specify=off  Q_nominal_unit=W  Q_nominal_value=1
  Thermal Mass2 : fl_lib/Thermal/Thermal Elements/Thermal Mass  mass=N2O_Rocket_Tank_Mass kg  sp_heat=N2O_Rocket_Tank_C J/(K*kg)  num_ports=foundation.enum.numPorts2.one  T_specify=on  T_priority=Low  T=Outside_temperature degC  T_nominal_specify=off  T_nominal_unit=K  T_nominal_value=1  Q_specify=off  Q_priority=None  Q=0 W  Q_nominal_specify=off  Q_nominal_unit=W  Q_nominal_value=1
  Output : Outport
  Output1 : Outport  Port=2
  Output2 : Outport  Port=3
  wires:
  PS-Simulink Converter1/1 -> Gain2/1
  PS-Simulink Converter/1 -> Gain3/1
  Gain3/1 -> Output1/1, Scope2/1
  Input1/1 -> Simulink-PS Converter1/1
  Input/1 -> Simulink-PS Converter/1
  Gain2/1 -> Output/1, Scope2/2
  Sum1/1 -> Scope1/1
  PS-Simulink Converter5/1 -> Sum1/1
  Constant/1 -> Sum1/2, Sum/2
  Sum/1 -> Scope1/2
  PS-Simulink Converter4/1 -> Sum/1
  PS-Simulink Converter2/1 -> Gain1/1
  Gain1/1 -> Scope/1, Output2/1
  Input2/1 -> Simulink-PS Converter3/1
  Input3/1 -> Simulink-PS Converter2/1
  connections:
  Pipe (G)9/RConn1 -- Pipe (G)/LConn1
  PS-Simulink Converter/LConn1 -- Pressure & Temperature Sensor (G)1/RConn2
  Pressure & Temperature Sensor (G)/LConn1 -- Pipe (G)8/RConn1 -- Constant Volume Chamber (G)1/LConn1
  Pipe (G)/RConn1 -- Local Restriction (G)/LConn1
  Pipe (G)4/LConn1 -- Pipe (G)1/RConn1 -- Pipe (G)2/LConn1
  Pipe (G)2/RConn1 -- Pipe (G)3/LConn1
  Pipe (G)1/LConn1 -- Local Restriction (G)/RConn1
  PS-Simulink Converter1/LConn1 -- Pressure & Temperature Sensor (G)/RConn2
  Simulink-PS Converter/RConn1 -- Local Restriction (G)/LConn2
  Simulink-PS Converter1/RConn1 -- Local Restriction (G)1/LConn2
  Reservoir (G)1/LConn1 -- Pressure & Temperature Sensor (G)/RConn1
  Pressure & Temperature Sensor (G)1/RConn1 -- Reservoir (G)2/LConn1
  PS-Simulink Converter4/LConn1 -- Pressure & Temperature Sensor (G)/RConn3
  Pressure & Temperature Sensor (G)1/RConn3 -- PS-Simulink Converter5/LConn1
  Local Restriction (G)2/LConn1 -- Pipe (G)5/RConn1
  Simulink-PS Converter2/RConn1 -- Local Restriction (G)2/LConn2
  Simulink-PS Converter3/RConn1 -- Local Restriction (G)3/LConn2
  Local Restriction (G)2/RConn1 -- Local Restriction (G)3/LConn1 -- Pipe (G)7/LConn1
  Convective Heat Transfer15/LConn1 -- Pipe (G)6/LConn2
  Constant Volume Chamber (G)2/LConn1 -- Pipe (G)7/RConn1 -- Pressure & Temperature Sensor (G)2/LConn1
  Pipe (G)8/LConn1 -- Pipe (G)3/RConn1
  Reservoir (G)/LConn1 -- Pipe (G)10/RConn1
  Solver Configuration/RConn1 -- Pressure & Temperature Sensor (G)1/LConn1 -- Pipe (G)9/LConn1 -- Constant Volume Chamber (G)/LConn1 -- Gas Properties (G)/RConn1
  Pipe (G)5/LConn1 -- Constant Volume Chamber (G)1/RConn1
  Pipe (G)9/LConn2 -- Convective Heat Transfer/LConn1
  Convective Heat Transfer1/LConn1 -- Pipe (G)/LConn2
  Pipe (G)2/LConn2 -- Convective Heat Transfer4/LConn1
  Pipe (G)3/LConn2 -- Convective Heat Transfer5/LConn1
  Convective Heat Transfer6/LConn1 -- Pipe (G)8/LConn2
  Convective Heat Transfer8/LConn1 -- Pipe (G)5/LConn2
  Convective Heat Transfer1/RConn1 -- Convective Heat Transfer11/RConn1 -- Convective Heat Transfer7/RConn1 -- Convective Heat Transfer14/RConn1 -- Convective Heat Transfer15/RConn1 -- Temperature Source9/LConn1 -- Convective Heat Transfer9/RConn1 -- Convective Heat Transfer8/RConn1 -- Convective Heat Transfer13/RConn1 -- Convective Heat Transfer6/RConn1 -- Convective Heat Transfer5/RConn1 -- Convective Heat Transfer4/RConn1 -- Convective Heat Transfer/RConn1 -- Convective Heat Transfer3/RConn1 -- Convective Heat Transfer2/RConn1
  Convective Heat Transfer9/LConn1 -- Pipe (G)7/LConn2
  Constant Volume Chamber (G)/LConn2 -- Convective Heat Transfer10/LConn1
  Thermal Mass/LConn1 -- Convective Heat Transfer11/LConn1 -- Convective Heat Transfer10/RConn1
  Constant Volume Chamber (G)1/LConn2 -- Convective Heat Transfer12/LConn1
  Convective Heat Transfer13/LConn1 -- Thermal Mass1/LConn1 -- Convective Heat Transfer12/RConn1
  Convective Heat Transfer2/LConn1 -- Pipe (G)1/LConn2
  Convective Heat Transfer14/LConn1 -- Thermal Mass2/LConn1 -- Convective Heat Transfer16/RConn1
  Reservoir (G)4/LConn1 -- Pressure & Temperature Sensor (G)2/RConn1
  PS-Simulink Converter2/LConn1 -- Pressure & Temperature Sensor (G)2/RConn2
  Convective Heat Transfer16/LConn1 -- Constant Volume Chamber (G)2/LConn2
  Pipe (G)6/RConn1 -- Reservoir (G)3/LConn1
  Local Restriction (G)3/RConn1 -- Pipe (G)6/LConn1
  Convective Heat Transfer3/LConn1 -- Pipe (G)4/LConn2
  Convective Heat Transfer7/LConn1 -- Pipe (G)10/LConn2
  Local Restriction (G)1/RConn1 -- Pipe (G)10/LConn1
  Local Restriction (G)1/LConn1 -- Pipe (G)4/RConn1

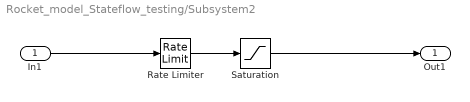
== system Rocket_model_Stateflow_testing/Subsystem2 ==
  In1 : Inport
  Rate Limiter : RateLimiter  RisingSlewLimit=2  FallingSlewLimit=-2
  Saturation : Saturate  UpperLimit=1  LowerLimit=0.0001
  Out1 : Outport
  wires:
  In1/1 -> Rate Limiter/1
  Rate Limiter/1 -> Saturation/1
  Saturation/1 -> Out1/1

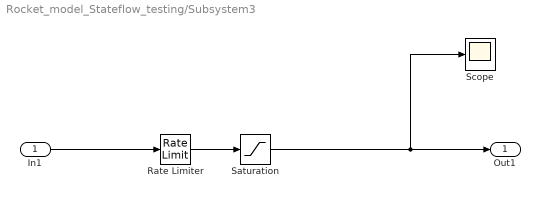
== system Rocket_model_Stateflow_testing/Subsystem3 ==
  In1 : Inport
  Rate Limiter : RateLimiter  RisingSlewLimit=2  FallingSlewLimit=-2
  Saturation : Saturate  UpperLimit=1  LowerLimit=0.0001
  Scope : Scope
  Out1 : Outport
  wires:
  In1/1 -> Rate Limiter/1
  Rate Limiter/1 -> Saturation/1
  Saturation/1 -> Scope/1, Out1/1

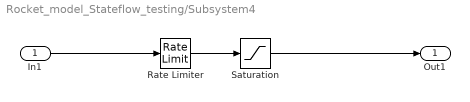
== system Rocket_model_Stateflow_testing/Subsystem4 ==
  In1 : Inport
  Rate Limiter : RateLimiter  RisingSlewLimit=2  FallingSlewLimit=-2
  Saturation : Saturate  UpperLimit=1  LowerLimit=0.0001
  Out1 : Outport
  wires:
  In1/1 -> Rate Limiter/1
  Rate Limiter/1 -> Saturation/1
  Saturation/1 -> Out1/1

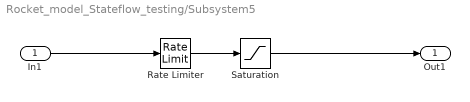
== system Rocket_model_Stateflow_testing/Subsystem5 ==
  In1 : Inport
  Rate Limiter : RateLimiter  RisingSlewLimit=2  FallingSlewLimit=-2
  Saturation : Saturate  UpperLimit=1  LowerLimit=0.0001
  Out1 : Outport
  wires:
  In1/1 -> Rate Limiter/1
  Rate Limiter/1 -> Saturation/1
  Saturation/1 -> Out1/1

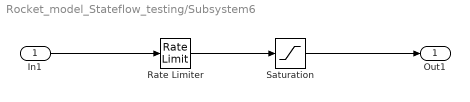
== system Rocket_model_Stateflow_testing/Subsystem6 ==
  In1 : Inport
  Rate Limiter : RateLimiter  RisingSlewLimit=2  FallingSlewLimit=-2
  Saturation : Saturate  UpperLimit=1  LowerLimit=0.0001
  Out1 : Outport
  wires:
  In1/1 -> Rate Limiter/1
  Rate Limiter/1 -> Saturation/1
  Saturation/1 -> Out1/1

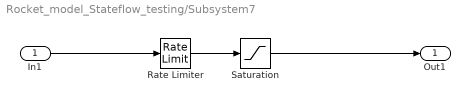
== system Rocket_model_Stateflow_testing/Subsystem7 ==
  In1 : Inport
  Rate Limiter : RateLimiter  RisingSlewLimit=2  FallingSlewLimit=-2
  Saturation : Saturate  UpperLimit=1  LowerLimit=0.0001
  Out1 : Outport
  wires:
  In1/1 -> Rate Limiter/1
  Rate Limiter/1 -> Saturation/1
  Saturation/1 -> Out1/1

== matlab function Rocket_model_Stateflow_testing/MATLAB Function1 ==
  data: u input; Curr_loop output; IO_2 output; IO_3 output; workspace input
function [Curr_loop, IO_2, IO_3]= fcn(u, workspace)

Curr_loop = uint8(zeros(1,69));
IO_2 = uint8(zeros(1,69));
IO_3 = uint8(zeros(1,69));

%Pressure sensor data conversion
press_sensor100bar_conv = @(x) (x - workspace.PT5302_OFFSET)/workspace.PT5302_GAIN;
press_sensor300bar_conv = @(x) (x - workspace.PT5500_OFFSET)/workspace.PT5500_GAIN;

%CurrentLoop message build
Curr_loop(1) = workspace.ID_RECEIVE;
Curr_loop(2) = workspace.PL_RECEIVE;
Curr_loop(3) = workspace.MSG_ID_RECEIVE;
Curr_loop(4) = workspace.CARDID_CURRENT_LOOP;
Curr_loop(5) = workspace.CARD_CURRENT_LOOP_SLOT;
Curr_loop_message = zeros(1,16);
Curr_loop_message(workspace.Low_p_ind) = press_sensor100bar_conv(u(3));   
Curr_loop_message(workspace.High_p_ind) = press_sensor300bar_conv(u(1));       
Curr_loop_message(workspace.GSE_Pressurizer_p_ind) = press_sensor300bar_conv(u(2));  
Curr_loop_message(workspace.GSE_oxidiser_p_ind) = press_sensor100bar_conv(60);
Curr_loop_message(workspace.N2O_fuel_level_ind) = u(4);
Curr_loop(6:end) = typecast(uint32(Curr_loop_message), 'uint8');

%IOcard2 message build
IO_2(1) = workspace.ID_RECEIVE;
IO_2(2) = workspace.PL_RECEIVE;
IO_2(3) = workspace.MSG_ID_RECEIVE;
IO_2(4) = workspace.CARDID_IO;
IO_2(5) = workspace.CARD_IO2_SLOT;
IO_2(5 + workspace.H0_bridge_state_ind) = 0;
IO_2(5 + workspace.H1_bridge_state_ind) = u(5);
IO_2(5 + workspace.H2_bridge_state_ind) = u(9);
IO_2(5 + workspace.H0_bridge_fault_state_ind) = 0;
IO_2(5 + workspace.H1_bridge_fault_state_ind) = 0;
IO_2(5 + workspace.H2_bridge_fault_state_ind) = 0;
IO_2(5 + workspace.Servo_0_state_ind) = u(7);
IO_2(5 + workspace.Servo_1_state_ind) = u(8);

%IOcard3 message build
IO_3(1) = workspace.ID_RECEIVE;
IO_3(2) = workspace.PL_RECEIVE;
IO_3(3) = workspace.MSG_ID_RECEIVE;
IO_3(4) = workspace.CARDID_IO;
IO_3(5) = workspace.CARD_IO3_SLOT;
IO_3(5 + workspace.H0_bridge_state_ind) = 0;
IO_3(5 + workspace.H1_bridge_state_ind) = u(6);
IO_3(5 + workspace.H2_bridge_state_ind) = u(10);
IO_3(5 + workspace.H0_bridge_fault_state_ind) = 0;
IO_3(5 + workspace.H1_bridge_fault_state_ind) = 0;
IO_3(5 + workspace.H2_bridge_fault_state_ind) = 0;

end

== matlab function Rocket_model_Stateflow_testing/Subsystem/MATLAB Function ==
  data: u input; prev input; workspace input; y output size=[1 4]
function y = fcn(u, prev, workspace)

y = zeros(1,4);
y = prev;
temp = u.';

if temp == workspace.N2O_fill_valve_open
    y(1) = 1;
elseif temp == workspace.N2O_fill_valve_close
    y(1) = 0;
end

if temp == workspace.Low_servo_open
    y(2) = 1;
elseif temp == workspace.Low_servo_close
    y(2) = 0;
end

if temp == workspace.High_servo_open
    y(3) = 1;
elseif temp == workspace.High_servo_close
    y(3) = 0;
end

if temp == workspace.N2_fill_valve_open
    y(4) = 1;
elseif temp == workspace.N2_fill_valve_close
    y(4) = 0;
end





% A = reshape(u, [workspace.UDP_GSE_send_packet_length, 4]).';
% 
% 
% if A(1,:) == workspace.N2_fill_valve_open
%     y(4) = 3.8e-5;
% elseif A(1,:) == workspace.N2_fill_valve_close
%     y(4) = 1e-10;
% end
% 
% if A(2,:) == workspace.High_servo_open
%     y(2) = 3.8e-5;
% elseif A(2,:) == workspace.High_servo_close
%     y(2) = 1e-10;
% end
% 
% if A(3,:) == workspace.Low_servo_open
%     y(3) = 3.8e-5;
% elseif A(2,:) == workspace.Low_servo_close
%     y(3) = 1e-10;
% end
% 
% if A(4,:) == workspace.N2O_fill_valve_open
%     y(1) = 3.8e-5;
% elseif A(4,:) == workspace.N2O_fill_valve_close
%     y(1) = 1e-10;
% end

end

== matlab function Rocket_model_Stateflow_testing/MATLAB Function2 ==
  data: u input; y output
function y = fcn(u)

y = zeros(1,6);

%N2 fill valve
if u(1) > 0.9
    y(1) = 0;
elseif u(1) < 0.1
    y(1) = 255;
else
    y(1) = 127;
end

%N2 release valve
if u(2) > 0.9
    y(2) = 0;
elseif u(2) < 0.1
    y(2) = 255;
else
    y(2) = 127;
end

%High servo
if u(3) > 0.9
    y(3) = 90;
elseif u(3) < 0.1
    y(3) = 0;
else
    y(3) = 45;
end

%Low servo
if u(4) > 0.9
    y(4) = 90;
elseif u(4) < 0.1
    y(4) = 0;
else
    y(4) = 45;
end

%N2O fill valve
if u(5) > 0.9
    y(5) = 0;
elseif u(5) < 0.1
    y(5) = 255;
else
    y(5) = 127;
end

%N2O release valve
if u(6) > 0.9
    y(6) = 0;
elseif u(6) < 0.1
    y(6) = 255;
else
    y(6) = 127;
end

end

== matlab function Rocket_model_Stateflow_testing/Subsystem1/MATLAB Function ==
  data: u input; workspace input; y output size=[1,2]; prev input size=[1,2]
function y = fcn(u, workspace, prev)

y = zeros(1,2);
y = prev;
temp = u.';

if temp == workspace.N2_release_valve_open 
    y(1) = 1;
elseif temp == workspace.N2_release_valve_close
    y(1) = 0;
end

if temp == workspace.N2O_release_valve_open 
    y(2) = 1;
elseif temp == workspace.N2O_release_valve_close
    y(2) = 0;
end





% A = reshape(u, [workspace.UDP_GSE_send_packet_length, 2]).';
% 
% if A(1,:) == workspace.N2_release_valve_open 
%     y(1) = 3.8e-5;
% elseif A(1,:) == workspace.N2_release_valve_close
%     y(1) = 1e-10;
% end
% 
% if A(2,:) == workspace.N2O_release_valve_open 
%     y(2) = 3.8e-5;
% elseif A(2,:) == workspace.N2O_release_valve_close
%     y(2) = 1e-10;
% end
